simulink model "cartpend_KunalJain_14AE10019"  (R2015a)
settings: Solver=ode45  StartTime=0.0  StopTime=10.0  RelTol=1e-3
libraries: simulink x2
settings Model: Creator=Aranya Dan  LastModifiedBy=Kunal

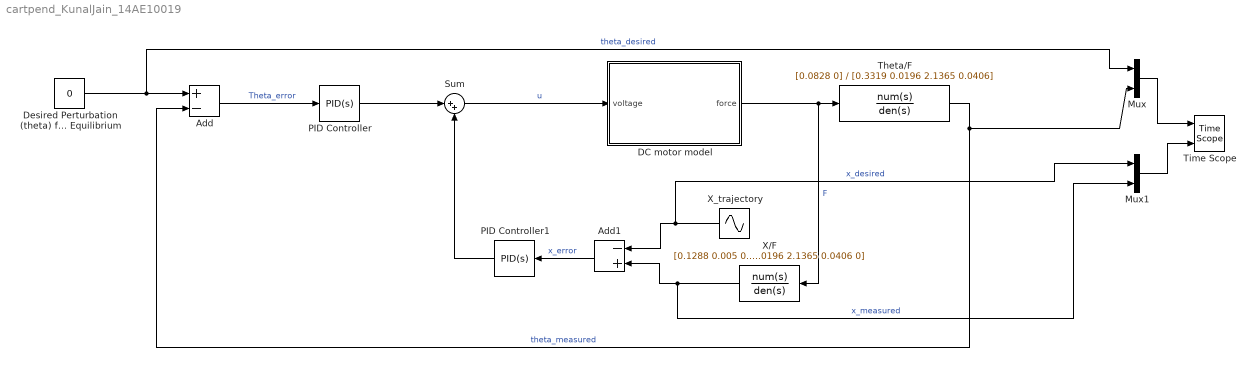
== system cartpend_KunalJain_14AE10019 ==
  Add : Sum  Inputs=+-
  Add1 : Sum  Inputs=-+
  DC motor model : Subsystem
  Desired Perturbation (theta) from Equilibrium : Constant  Value=0
  Mux : Mux  Inputs=2
  Mux1 : Mux  Inputs=2
  PID Controller : simulink/Continuous/PID Controller  Controller=PID  TimeDomain=Continuous-time  SampleTime=-1  IntegratorMethod=Forward Euler  FilterMethod=Forward Euler  Form=Parallel  UseFilter=on  ControllerParametersSource=internal  P=185.474230733501  I=0.149570338875648  D=826.40709745591  N=0.0504202201249579  InitialConditionSource=internal  InitialConditionForIntegrator=0  InitialConditionForFilter=0  ExternalReset=none  LimitOutput=off  UpperSaturationLimit=inf  LowerSaturationLimit=-inf  LinearizeAsGain=on  AntiWindupMode=none  Kb=1  TrackingMode=off  Kt=1  PParamMin=[]  PParamMax=[]  IParamMin=[]  IParamMax=[]  DParamMin=[]  DParamMax=[]  NParamMin=[]  NParamMax=[]  KbParamMin=[]  KbParamMax=[]  KtParamMin=[]  KtParamMax=[]  POutMin=[]  POutMax=[]  IOutMin=[]  IOutMax=[]  DOutMin=[]  DOutMax=[]  NOutMin=[]  NOutMax=[]  KbOutMin=[]  KbOutMax=[]  KtOutMin=[]  KtOutMax=[]  IntegratorOutMin=[]  IntegratorOutMax=[]  FilterOutMin=[]  FilterOutMax=[]  SumOutMin=[]  SumOutMax=[]  SumI1OutMin=[]  SumI1OutMax=[]  SumI2OutMin=[]  SumI2OutMax=[]  SumI3OutMin=[]  SumI3OutMax=[]  SumDOutMin=[]  SumDOutMax=[]  SaturationOutMin=[]  SaturationOutMax=[]  IntegratorContinuousStateAttributes=''  IntegratorStateMustResolveToSignalObject=off  IntegratorRTWStateStorageClass=Auto  FilterContinuousStateAttributes=''  FilterStateMustResolveToSignalObject=off  FilterRTWStateStorageClass=Auto  DifferentiatorICPrevScaledInput=0  DifferentiatorOutMin=[]  DifferentiatorOutMax=[]
  PID Controller1 : simulink/Continuous/PID Controller  Controller=PID  TimeDomain=Continuous-time  SampleTime=-1  IntegratorMethod=Forward Euler  FilterMethod=Forward Euler  Form=Parallel  UseFilter=on  ControllerParametersSource=internal  P=831.140160718589  I=29249.2650914478  D=5.88987419538334  N=29549.3786820731  InitialConditionSource=internal  InitialConditionForIntegrator=0  InitialConditionForFilter=0  ExternalReset=none  LimitOutput=off  UpperSaturationLimit=inf  LowerSaturationLimit=-inf  LinearizeAsGain=on  AntiWindupMode=none  Kb=1  TrackingMode=off  Kt=1  PParamMin=[]  PParamMax=[]  IParamMin=[]  IParamMax=[]  DParamMin=[]  DParamMax=[]  NParamMin=[]  NParamMax=[]  KbParamMin=[]  KbParamMax=[]  KtParamMin=[]  KtParamMax=[]  POutMin=[]  POutMax=[]  IOutMin=[]  IOutMax=[]  DOutMin=[]  DOutMax=[]  NOutMin=[]  NOutMax=[]  KbOutMin=[]  KbOutMax=[]  KtOutMin=[]  KtOutMax=[]  IntegratorOutMin=[]  IntegratorOutMax=[]  FilterOutMin=[]  FilterOutMax=[]  SumOutMin=[]  SumOutMax=[]  SumI1OutMin=[]  SumI1OutMax=[]  SumI2OutMin=[]  SumI2OutMax=[]  SumI3OutMin=[]  SumI3OutMax=[]  SumDOutMin=[]  SumDOutMax=[]  SaturationOutMin=[]  SaturationOutMax=[]  IntegratorContinuousStateAttributes=''  IntegratorStateMustResolveToSignalObject=off  IntegratorRTWStateStorageClass=Auto  FilterContinuousStateAttributes=''  FilterStateMustResolveToSignalObject=off  FilterRTWStateStorageClass=Auto  DifferentiatorICPrevScaledInput=0  DifferentiatorOutMin=[]  DifferentiatorOutMax=[]
  Sum : Sum  Inputs=|++
  Theta/F : TransferFcn  Numerator=[0.0828 0]  Denominator=[0.3319 0.0196 2.1365 0.0406]
  Time Scope : TimeScope  DefaultConfigurationName=spbscopes.TimeScopeBlockCfg  NumInputPorts=2
  X/F : TransferFcn  Numerator=[0.1288 0.005 0.8123]  Denominator=[0.3319 0.0196 2.1365 0.0406 0]
  X_trajectory : Sin  Amplitude=0.2  SampleTime=0
  wires:
  DC motor model/1(force) -> Theta/F/1, X/F/1  "F"
  Theta/F/1 -> Mux/2, Add/2  "theta_measured"
  Sum/1 -> DC motor model/1(voltage)  "u"
  Add/1 -> PID Controller/1  "Theta_error"
  X_trajectory/1 -> Mux1/1, Add1/1  "x_desired"
  X/F/1 -> Mux1/2, Add1/2  "x_measured"
  Add1/1 -> PID Controller1/1  "x_error"
  Desired Perturbation (theta) from Equilibrium/1 -> Mux/1, Add/1  "theta_desired"
  PID Controller/1 -> Sum/1
  Mux/1 -> Time Scope/1
  Mux1/1 -> Time Scope/2
  PID Controller1/1 -> Sum/2

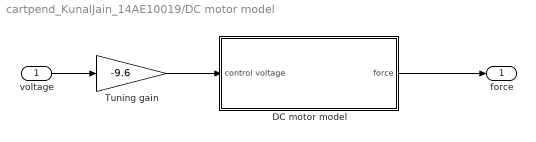
== system cartpend_KunalJain_14AE10019/DC motor model ==
  voltage : Inport
  DC motor model : Subsystem  mask{J=0.0000140, Kt=0.05, Kb=0.05, d=0.000001, R=2.5, L=0.0025}
      mask prompts: J "Moment of inertia"; Kt "Torque constant"; Kb "Electromotive force constant"; d "Linear approximation of viscous friction"; R "Electrical circuit resistance"; L "Electrical circuit inductance"
      mask Display: disp('DC motor')
  Tuning gain : Gain  Gain=-9.6
  force : Outport
  wires:
  Tuning gain/1 -> DC motor model/1(control voltage)
  voltage/1 -> Tuning gain/1
  DC motor model/1(force) -> force/1

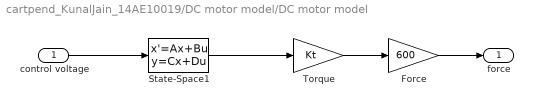
== system cartpend_KunalJain_14AE10019/DC motor model/DC motor model ==
  control voltage : Inport
  Force : Gain  Gain=600
  State-Space1 : StateSpace  A=[-d/J Kt/J;-Kb/L -R/L]  B=[0; 1/L]  C=[0 1]  D=0  X0=0
  Torque : Gain  Gain=Kt
  force : Outport
  wires:
  control voltage/1 -> State-Space1/1
  State-Space1/1 -> Torque/1
  Torque/1 -> Force/1
  Force/1 -> force/1
